simulink model "OES_compatible"  (R2017b)
settings: configuration reference "Configuration" (kept outside this file)
undefined symbols (not defined in the file or in its folder): sats
settings Model: Creator=Ethan  LastModifiedBy=Ethan
settings ConfigSetRef: SourceLocation=Base Workspace

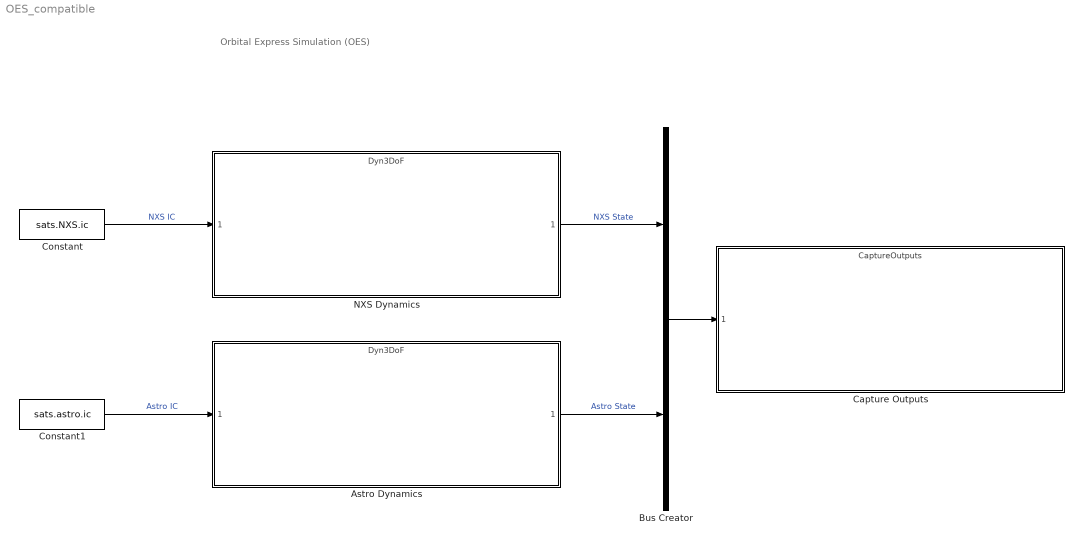
== system OES_compatible ==
  note: Orbital Express Simulation (OES)
  Astro Dynamics : ModelReference  ModelNameDialog=Dyn3DoF.slx  ParameterArgumentNames=CON  ParameterArgumentValues=CON  UsingDefaultArgumentValue=0  ModelReferenceVersion=1.36
  Bus Creator : BusCreator  Inputs=2  OutDataTypeStr=Bus: Bus_outputs  NonVirtualBus=on
      settings: InheritFromInputs=off
  Capture Outputs : ModelReference  ModelNameDialog=CaptureOutputs.slx  SimulationMode=Normal  ModelReferenceVersion=1.24
  Constant : Constant  Value=sats.NXS.ic  OutDataTypeStr=Bus: Bus_state
  Constant1 : Constant  Value=sats.astro.ic  OutDataTypeStr=Bus: Bus_state
  NXS Dynamics : ModelReference  ModelNameDialog=Dyn3DoF.slx  ParameterArgumentNames=CON  ParameterArgumentValues=CON  UsingDefaultArgumentValue=0  ModelReferenceVersion=1.36
  wires:
  Constant/1 -> NXS Dynamics/1  "NXS IC"
  Constant1/1 -> Astro Dynamics/1  "Astro IC"
  Astro Dynamics/1 -> Bus Creator/2  "Astro State"
  NXS Dynamics/1 -> Bus Creator/1  "NXS State"
  Bus Creator/1 -> Capture Outputs/1
